simulink model "PSO_1"  (R2021a)
settings: Solver=FixedStepAuto  StartTime=0.0  StopTime=3  FixedStep=5e-05  RelTol=1e-3  EnableMultiTasking=on
libraries: spsIGBTDiodeLib x6, powerlib_extras x3, simulink x2, spsCurrentMeasurementLib x1, spsDCVoltageSourceLib x1, spsPermanentMagnetSynchronousMachineLib x1, spspowerguiLib x1
settings Model: Creator=nit  LastModifiedBy=DELL
settings SolverCC: AlgebraicLoopSolver=TrustRegion
settings DataIOCC: LimitDataPoints=on  SaveFormat=Array  ReturnWorkspaceOutputs=off
settings OptimizationCC: LifeSpan=inf
settings DebuggingCC: SolverPrmCheckMsg=warning  SFUnexpectedBacktrackingDiag=warning  SFNoUnconditionalDefaultTransitionDiag=warning  SFExecutionAtInitializationDiag=none  SFMachineParentedDataDiag=warning  ArithmeticOperatorsInVariantConditions=warning
settings HardwareCC: ProdBitPerPointer=32  ProdBitPerSizeT=32  ProdBitPerPtrDiffT=32  ProdLargestAtomicFloat=None  ProdIntDivRoundTo=Undefined  ProdEndianess=Unspecified  ProdWordSize=32  ProdHWDeviceType=32-bit Generic
settings ModelReferenceCC: PropagateSignalLabelsOutOfModel=off
settings SFSimCC: SimUseLocalCustomCode=off  CustomCodeUndefinedFunction=UseInterfaceOnly
settings RTWCC: RTWUseLocalCustomCode=off
settings CodeAppCC: StateflowObjectComments=on
settings GRTTargetCC: TargetLangStandard=C89/C90 (ANSI)
settings ConfigComp: CovMetricSettings=dw  CovSaveCumulativeToWorkspaceVar=on  CovSaveSingleToWorkspaceVar=on  CovExternalEMLEnable=off  CovSFcnEnable=off
settings SimscapeCC: SimscapeNormalizeSystem=off
settings ConfigurationSet: Description=SimMechanics 2G

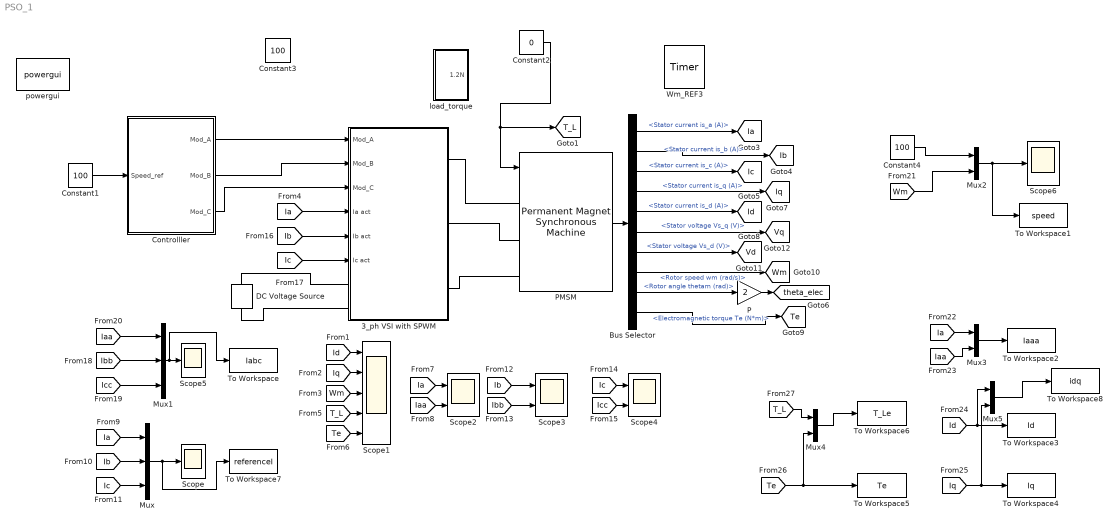
== system PSO_1 ==
  3_ph VSI with SPWM : Subsystem
  Bus Selector : BusSelector  OutputSignals=Stator current is_a (A),Stator current is_b (A),Stator current is_c (A),Stator current is_q (A),Stator current is_d (A),Stator voltage Vs_q (V),Stator voltage Vs_d (V),Rotor speed wm (rad/s),Rotor angle thetam (rad),Electromagnetic torque Te (N*m)
  Constant1 : Constant  Value=100
  Constant2 : Constant  Value=0
  Constant3 : Constant  Value=100
  Constant4 : Constant  Value=100
  Controlller : Subsystem
  DC Voltage Source : spsDCVoltageSourceLib/DC Voltage Source  Amplitude=100  Measurements=None
  Mux : Mux  Inputs=3
  Mux1 : Mux  Inputs=3
  Mux{2..5} (4 alike) : Mux  Inputs=2
  P : Gain  Gain=2
  PMSM : spsPermanentMagnetSynchronousMachineLib/Permanent Magnet Synchronous Machine  NbPhases=3  FluxDistribution=Sinusoidal  RotorType=Salient-pole  MechanicalLoad=Torque Tm  PresetModel=No  ShowDetailedParameters=on  MeasurementBus=off  Resistance=0.18  Inductance=8.5e-3  dqInductances=[0.0125,0.0057]  La=0.000835  MachineConstant=Flux linkage established by magnets (V.s)  Flux=0.123  VoltageCst=44.6195  TorqueCst=0.369  Flat=120  Mechanical=[0.00062 0.0003035 2 0]  PolePairs=2  InitialConditions=[0,0, 0,0]  InitialConditions5ph=[0 0 0 0 0 0]  RefAngle=Aligned with phase A axis (original Park)  IterativeDiscreteModel=Trapezoidal non iterative  TsBlock=-1  TsPowergui=0
  Scope : Scope
  Scope1 : Scope  NumInputPorts=5
  Scope2 : Scope  NumInputPorts=2
  Scope3 : Scope  NumInputPorts=2
  Scope4 : Scope  NumInputPorts=2
  Scope5 : Scope
  Scope6 : Scope
  To Workspace : ToWorkspace  VariableName=Iabc  SaveFormat=Timeseries  SampleTime=-1
  To Workspace1 : ToWorkspace  VariableName=speed  SaveFormat=Timeseries  SampleTime=-1
  To Workspace2 : ToWorkspace  VariableName=Iaaa  SaveFormat=Timeseries  SampleTime=-1
  To Workspace3 : ToWorkspace  VariableName=Id  SaveFormat=Timeseries  SampleTime=-1
  To Workspace4 : ToWorkspace  VariableName=Iq  SaveFormat=Timeseries  SampleTime=-1
  To Workspace5 : ToWorkspace  VariableName=Te  SaveFormat=Timeseries  SampleTime=-1
  To Workspace6 : ToWorkspace  VariableName=T_Le  SaveFormat=Timeseries  SampleTime=-1
  To Workspace7 : ToWorkspace  VariableName=referenceI  SaveFormat=Timeseries  SampleTime=-1
  To Workspace8 : ToWorkspace  VariableName=idq  SaveFormat=Timeseries  SampleTime=-1
  Wm_REF3 : powerlib_extras/Control  Blocks/Timer  t="[ 0 0.08  0.5 ]"  e=[100 80 200]
      settings: SourceProductBaseCode=PS
  load_torque : Subsystem
  powergui : spspowerguiLib/powergui  Priority=1  SimulationMode=Discrete  SampleTime=50e-6  frequency=60  Iterations=50  frequencyindice=0  Pbase=100e6  ErrMax=1e-4  UnitsV=kV  UnitsW=MW  buscounter=0  FunctionMessages=off  echomessages=off  EnableUseOfTLC=off  CurrentSourceSwitches=off  DisableSnubberDevices=off  DisableRonSwitches=off  DisableVfSwitches=off  DisplayEquations=off  AutomaticDiscreteSolvers=off  SolverType=Tustin  Interpol=off  ExternalGateDelay=off  methode=off  Ts=0  x0status=blocks  SPID=off  SwTol=0  HookPort=off  NonlinearTolerance=1e-4  nMaxIteration=100  ContinueOnMaxIteration=off  RestoreLinks=warning  ResistiveCurrentMeasurement=off  Frange=[0:2:500]  Ylog=off  Xlog=on  ShowGrid=off  save=off  variable=ZData  structure=0  ZoomFFT=off  StartTime=0.0  cycles=1  DisplayStyle=1  fundamental=60  FreqAxis=off  MaxFrequency=1000  frequencyindicesteady=1  RmsSteady=1  display=off
  tag scope: Ia=global, Ib=global, Ic=global, Id=global, Iq=global, T_L=global, Te=global, Vd=global, Vq=global, Wm=global, theta_elec=global
  wires:
  PMSM/1 -> Bus Selector/1
  Bus Selector/5 -> [Id]  "<Stator current is_d (A)>"
  Bus Selector/4 -> [Iq]  "<Stator current is_q (A)>"
  Bus Selector/3 -> [Ic]  "<Stator current is_c (A)>"
  Bus Selector/2 -> [Ib]  "<Stator current is_b (A)>"
  Bus Selector/1 -> [Ia]  "<Stator current is_a (A)>"
  Bus Selector/9 -> P/1  "<Rotor angle thetam (rad)>"
  P/1 -> [theta_elec]
  Controlller/1(Mod_A) -> 3_ph VSI with SPWM/1(Mod_A)
  Controlller/2(Mod_B) -> 3_ph VSI with SPWM/2(Mod_B)
  Controlller/3(Mod_C) -> 3_ph VSI with SPWM/3(Mod_C)
  Bus Selector/10 -> [Te]  "<Electromagnetic torque Te (N*m)>"
  Bus Selector/8 -> [Wm]  "<Rotor speed wm (rad/s)>"
  Bus Selector/7 -> [Vd]  "<Stator voltage Vs_d (V)>"
  Bus Selector/6 -> [Vq]  "<Stator voltage Vs_q (V)>"
  [Id] -> Scope1/1
  [Te] -> Scope1/5
  [T_L] -> Scope1/4
  [Wm] -> Scope1/3
  [Iq] -> Scope1/2
  Constant1/1 -> Controlller/1(Speed_ref)
  [Ia] -> Scope2/1
  [Iaa] -> Scope2/2
  [Ib] -> Scope3/1
  [Ibb] -> Scope3/2
  [Ic] -> Scope4/1
  [Icc] -> Scope4/2
  [Ia] -> 3_ph VSI with SPWM/4(Ia act)
  [Ib] -> 3_ph VSI with SPWM/5(Ib act)
  [Ic] -> 3_ph VSI with SPWM/6(Ic act)
  [Ia] -> Mux/1
  [Ib] -> Mux/2
  [Ic] -> Mux/3
  Mux/1 -> To Workspace7/1, Scope/1
  [Iaa] -> Mux1/1
  [Ibb] -> Mux1/2
  [Icc] -> Mux1/3
  Mux1/1 -> To Workspace/1, Scope5/1
  Mux2/1 -> To Workspace1/1, Scope6/1
  Constant4/1 -> Mux2/1
  [Wm] -> Mux2/2
  [Ia] -> Mux3/1
  [Iaa] -> Mux3/2
  Mux3/1 -> To Workspace2/1
  [Id] -> Mux5/1, To Workspace3/1
  [Iq] -> Mux5/2, To Workspace4/1
  [Te] -> Mux4/2, To Workspace5/1
  [T_L] -> Mux4/1
  Mux4/1 -> To Workspace6/1
  Mux5/1 -> To Workspace8/1
  Constant2/1 -> [T_L], PMSM/1
  connections:
  3_ph VSI with SPWM/LConn2 -- DC Voltage Source/LConn1
  PMSM/LConn2 -- 3_ph VSI with SPWM/RConn2
  3_ph VSI with SPWM/LConn1 -- DC Voltage Source/RConn1
  PMSM/LConn1 -- 3_ph VSI with SPWM/RConn1
  3_ph VSI with SPWM/RConn3 -- PMSM/LConn3

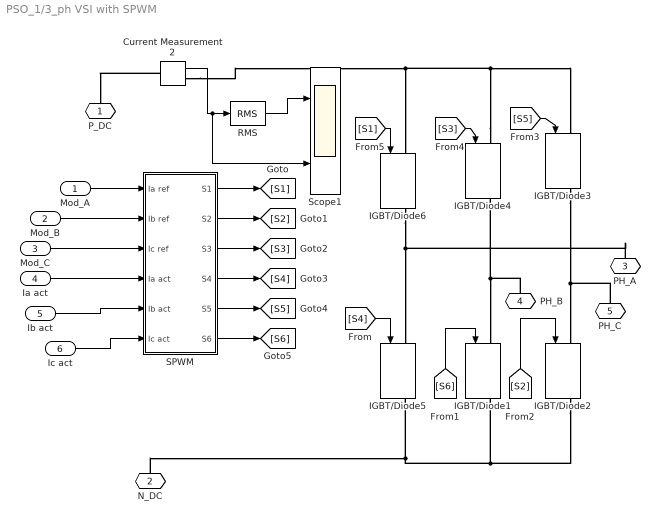
== system PSO_1/3_ph VSI with SPWM ==
  Mod_A : Inport
  Mod_B : Inport  Port=2
  Mod_C : Inport  Port=3
  Ia act : Inport  Port=4
  Ib act : Inport  Port=5
  Ic act : Inport  Port=6
  Current Measurement2 : spsCurrentMeasurementLib/Current Measurement  PhasorSimulation=off  OutputType=Complex  PSBequivalent=0
  IGBT/Diode{1..6} (6 alike) : spsIGBTDiodeLib/IGBT//Diode  Ron=1e-3  Rs=1e5  Cs=inf  Measurements=on
  RMS : powerlib_extras/Measurements/RMS  f1=100
      settings: SourceProductBaseCode=PS
  SPWM : Subsystem
  Scope1 : Scope  NumInputPorts=2
  P_DC : PMIOPort  Side=Left
  N_DC : PMIOPort  Port=2  Side=Left
  PH_A : PMIOPort  Port=3  Side=Right
  PH_B : PMIOPort  Port=4  Side=Right
  PH_C : PMIOPort  Port=5  Side=Right
  wires:
  [S1] -> IGBT/Diode6/1
  [S3] -> IGBT/Diode4/1
  [S5] -> IGBT/Diode3/1
  [S4] -> IGBT/Diode5/1
  [S6] -> IGBT/Diode1/1
  [S2] -> IGBT/Diode2/1
  Current Measurement2/1 -> Scope1/2, RMS/1
  RMS/1 -> Scope1/1
  SPWM/1(S1) -> [S1]
  SPWM/2(S2) -> [S2]
  SPWM/3(S3) -> [S3]
  SPWM/4(S4) -> [S4]
  SPWM/5(S5) -> [S5]
  SPWM/6(S6) -> [S6]
  Mod_A/1 -> SPWM/1(Ia ref)
  Mod_B/1 -> SPWM/2(Ib ref)
  Mod_C/1 -> SPWM/3(Ic ref)
  Ia act/1 -> SPWM/4(Ia act)
  Ib act/1 -> SPWM/5(Ib act)
  Ic act/1 -> SPWM/6(Ic act)
  connections:
  PH_A/RConn1 -- IGBT/Diode5/LConn1 -- IGBT/Diode6/RConn1
  PH_B/RConn1 -- IGBT/Diode1/LConn1 -- IGBT/Diode4/RConn1
  IGBT/Diode3/RConn1 -- PH_C/RConn1 -- IGBT/Diode2/LConn1
  IGBT/Diode4/LConn1 -- IGBT/Diode3/LConn1 -- Current Measurement2/RConn1 -- IGBT/Diode6/LConn1
  N_DC/RConn1 -- IGBT/Diode1/RConn1 -- IGBT/Diode2/RConn1 -- IGBT/Diode5/RConn1
  Current Measurement2/LConn1 -- P_DC/RConn1

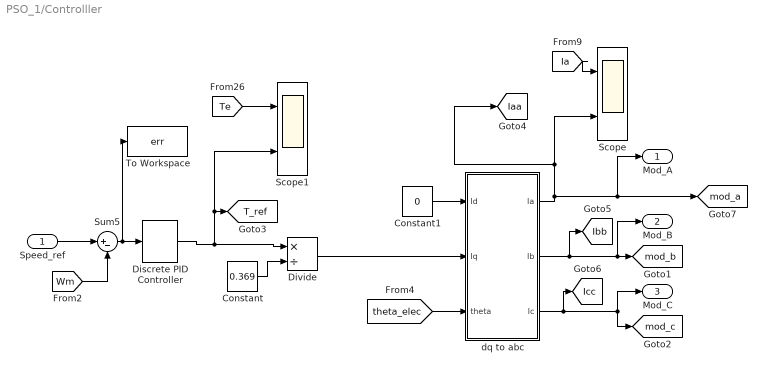
== system PSO_1/Controlller ==
  Speed_ref : Inport
  Constant : Constant  Value=0.369
  Constant1 : Constant  Value=0
  Discrete PID Controller : powerlib_extras/Discrete  Control Blocks/Discrete PID Controller  Kp=100  Ki=1  Kd=0  TcD=0  Par_Limits=[4 -4]  Init=0  Ts=5e-5
      settings: SourceProductBaseCode=PS
  Divide : Product  Inputs=*/
  Scope : Scope  NumInputPorts=2
  Scope1 : Scope  NumInputPorts=2
  Sum5 : Sum  Inputs=|+-
  To Workspace : ToWorkspace  VariableName=err  SaveFormat=Timeseries  SampleTime=-1
  dq to abc : MATLAB Function  TreatAsAtomicUnit=on
  Mod_A : Outport
  Mod_B : Outport  Port=2
  Mod_C : Outport  Port=3
  tag scope: Iaa=global, Ibb=global, Icc=global, T_ref=global, mod_a=global, mod_b=global, mod_c=global
  wires:
  [theta_elec] -> dq to abc/3(theta)
  Divide/1 -> dq to abc/2(Iq)
  dq to abc/1(Ia) -> [Iaa], Scope/2, Mod_A/1, [mod_a]
  dq to abc/2(Ib) -> [Ibb], Mod_B/1, [mod_b]
  Sum5/1 -> To Workspace/1, Discrete PID Controller/1
  Speed_ref/1 -> Sum5/1
  [Wm] -> Sum5/2
  Constant/1 -> Divide/2
  Discrete PID Controller/1 -> Divide/1, Scope1/2, [T_ref]
  Constant1/1 -> dq to abc/1(Id)
  [Ia] -> Scope/1
  dq to abc/3(Ic) -> [Icc], Mod_C/1, [mod_c]
  [Te] -> Scope1/1

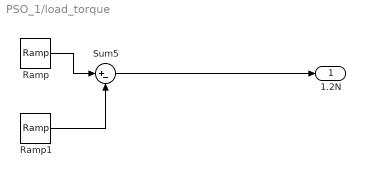
== system PSO_1/load_torque ==
  Ramp : simulink/Sources/Ramp  slope=3  start=0.4  InitialOutput=0
  Ramp1 : simulink/Sources/Ramp  slope=3  start=0.8  InitialOutput=0
  Sum5 : Sum  Inputs=|+-
  1.2N : Outport
  wires:
  Ramp1/1 -> Sum5/2
  Sum5/1 -> 1.2N/1
  Ramp/1 -> Sum5/1

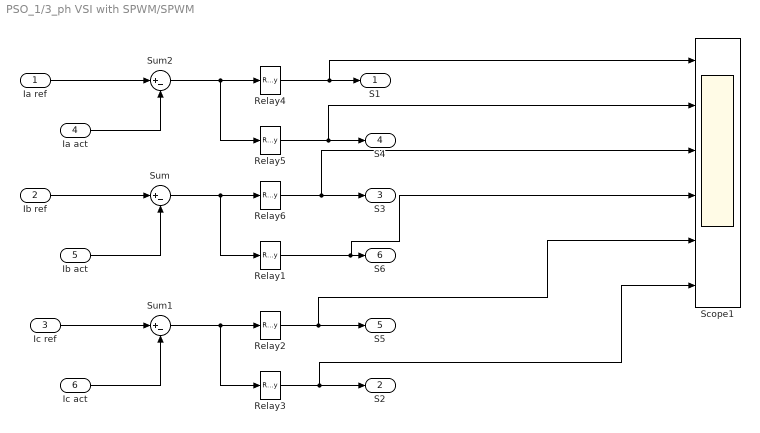
== system PSO_1/3_ph VSI with SPWM/SPWM ==
  Ia ref : Inport
  Ib ref : Inport  Port=2
  Ic ref : Inport  Port=3
  Ia act : Inport  Port=4
  Ib act : Inport  Port=5
  Ic act : Inport  Port=6
  Relay1 : Relay  OnSwitchValue=0.01  OffSwitchValue=-0.01  OnOutputValue=0  OffOutputValue=1
  Relay2 : Relay  OnSwitchValue=0.01  OffSwitchValue=-0.01
  Relay3 : Relay  OnSwitchValue=0.01  OffSwitchValue=-0.01  OnOutputValue=0  OffOutputValue=1
  Relay4 : Relay  OnSwitchValue=0.01  OffSwitchValue=-0.01
  Relay5 : Relay  OnSwitchValue=0.01  OffSwitchValue=-0.01  OnOutputValue=0  OffOutputValue=1
  Relay6 : Relay  OnSwitchValue=0.01  OffSwitchValue=-0.01
  Scope1 : Scope  NumInputPorts=6
  Sum : Sum  Inputs=|+-
  Sum1 : Sum  Inputs=|+-
  Sum2 : Sum  Inputs=|+-
  S1 : Outport
  S2 : Outport  Port=2
  S3 : Outport  Port=3
  S4 : Outport  Port=4
  S5 : Outport  Port=5
  S6 : Outport  Port=6
  wires:
  Sum/1 -> Relay1/1, Relay6/1
  Sum1/1 -> Relay3/1, Relay2/1
  Sum2/1 -> Relay5/1, Relay4/1
  Relay4/1 -> Scope1/1, S1/1
  Relay5/1 -> Scope1/2, S4/1
  Relay6/1 -> Scope1/3, S3/1
  Relay1/1 -> Scope1/4, S6/1
  Relay2/1 -> Scope1/5, S5/1
  Relay3/1 -> Scope1/6, S2/1
  Ia ref/1 -> Sum2/1
  Ia act/1 -> Sum2/2
  Ib ref/1 -> Sum/1
  Ib act/1 -> Sum/2
  Ic ref/1 -> Sum1/1
  Ic act/1 -> Sum1/2

== matlab function PSO_1/Controlller/dq to abc ==
  data: Id input; Iq input; Ia output; theta input; Ib output; Ic output
function [Ia,Ib,Ic]= fcn(Id, Iq, theta)
Ia = Id*cos(theta)- Iq*sin(theta)
Ib = Id*cos(theta-(2*pi/3))- Iq*sin(theta-(2*pi/3))
Ic = Id*cos(theta+(2*pi/3))- Iq*sin(theta+(2*pi/3))
